simulink model "Clarke_Transformation"  (R2020a)
settings: Solver=VariableStepAuto  StartTime=0.0  StopTime=2  RelTol=1e-3
libraries: powerlib_meascontrol x2
settings Model: Creator=ahmed  LastModifiedBy=ahmed
settings DataIOCC: Refine=250

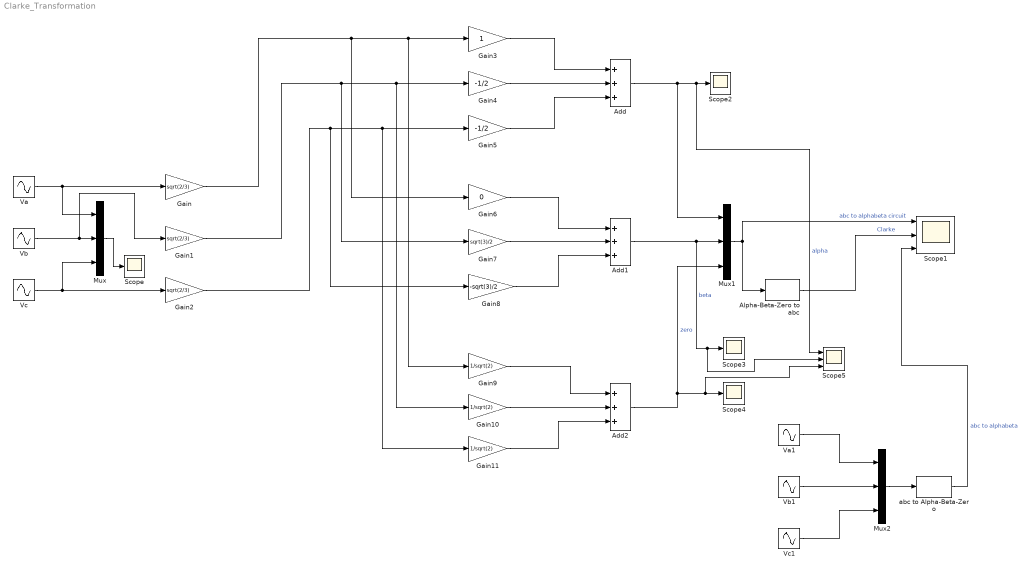
== system Clarke_Transformation ==
  Add : Sum  Inputs=+++
  Add1 : Sum  Inputs=+++
  Add2 : Sum  Inputs=+++
  Alpha-Beta-Zero to abc : powerlib_meascontrol/Transformations/Alpha-Beta-Zero to abc
      settings: SourceProductBaseCode=PS
  Gain : Gain  Gain=sqrt(2/3)
  Gain1 : Gain  Gain=sqrt(2/3)
  Gain10 : Gain  Gain=1/sqrt(2)
  Gain11 : Gain  Gain=1/sqrt(2)
  Gain2 : Gain  Gain=sqrt(2/3)
  Gain3 : Gain
  Gain4 : Gain  Gain=-1/2
  Gain5 : Gain  Gain=-1/2
  Gain6 : Gain  Gain=0
  Gain7 : Gain  Gain=sqrt(3)/2
  Gain8 : Gain  Gain=-sqrt(3)/2
  Gain9 : Gain  Gain=1/sqrt(2)
  Mux : Mux  Inputs=3
  Mux1 : Mux  Inputs=3
  Mux2 : Mux  Inputs=3
  Scope{,2..4} (4 alike) : Scope
  Scope1 : Scope  NumInputPorts=3
  Scope5 : Scope  NumInputPorts=3
  Va : Sin  Amplitude=10  Frequency=50  SampleTime=0
  Va1 : Sin  Amplitude=10  Frequency=50  SampleTime=0
  Vb : Sin  Amplitude=10  Frequency=50  Phase=120*(pi/180)  SampleTime=0
  Vb1 : Sin  Amplitude=10  Frequency=50  Phase=120*(pi/180)  SampleTime=0
  Vc : Sin  Amplitude=10  Frequency=50  Phase=240*(pi/180)  SampleTime=0
  Vc1 : Sin  Amplitude=10  Frequency=50  Phase=240*(pi/180)  SampleTime=0
  abc to Alpha-Beta-Zero : powerlib_meascontrol/Transformations/abc to Alpha-Beta-Zero
  wires:
  Va/1 -> Mux/1, Gain/1
  Vb/1 -> Gain1/1, Mux/2
  Vc/1 -> Mux/3, Gain2/1
  Mux/1 -> Scope/1
  Gain3/1 -> Add/1
  Gain5/1 -> Add/3
  Gain4/1 -> Add/2
  Gain7/1 -> Add1/2
  Gain6/1 -> Add1/1
  Gain8/1 -> Add1/3
  Gain9/1 -> Add2/1
  Gain10/1 -> Add2/2
  Gain11/1 -> Add2/3
  Add1/1 -> Scope5/2, Scope3/1, Mux1/2  "beta"
  Add/1 -> Mux1/1, Scope5/1, Scope2/1  "alpha"
  Add2/1 -> Scope5/3, Scope4/1, Mux1/3  "zero"
  Mux1/1 -> Alpha-Beta-Zero to abc/1, Scope1/1  "abc to alphabeta circuit"
  Alpha-Beta-Zero to abc/1 -> Scope1/2  "Clarke"
  Gain/1 -> Gain6/1, Gain9/1, Gain3/1
  Gain1/1 -> Gain7/1, Gain10/1, Gain4/1
  Gain2/1 -> Gain8/1, Gain11/1, Gain5/1
  Vb1/1 -> Mux2/2
  Va1/1 -> Mux2/1
  Vc1/1 -> Mux2/3
  Mux2/1 -> abc to Alpha-Beta-Zero/1
  abc to Alpha-Beta-Zero/1 -> Scope1/3  "abc to alphabeta"
